simulink model "toma_datos"  (R2023a)
settings: Solver=VariableStepAuto  StartTime=0.0  StopTime=10.0  RelTol=1e-3
libraries: daqlib x2
settings Model: Creator=Juan  LastModifiedBy=Juan

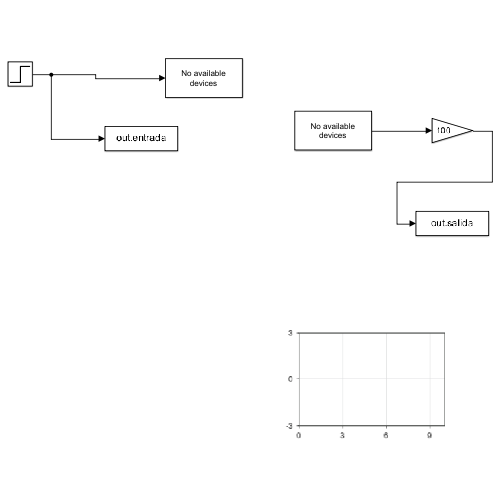
[thumbnail: Simulink's stored preview of the top-level diagram]
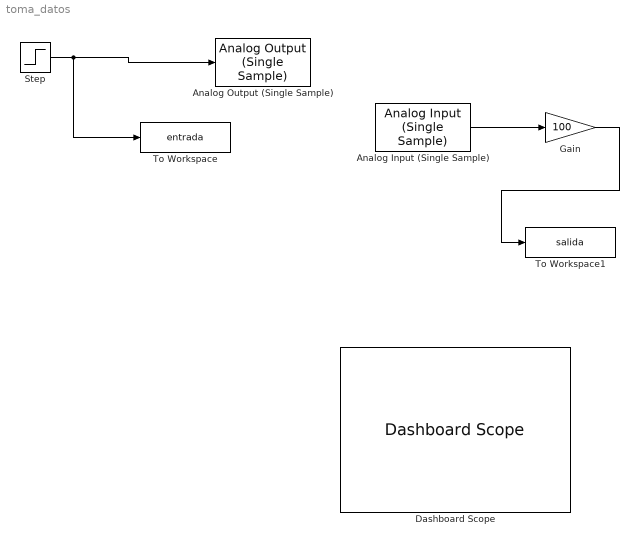
== system toma_datos ==
  Analog Input (Single Sample) : daqlib/Analog Input (Single Sample)  DeviceMenu=(none)  Device=(none)  BlockSampleTime=1  NChannelsSelected=1  NPorts=1 for all channels  OutputTimestamp=off
  Analog Output (Single Sample) : daqlib/Analog Output (Single Sample)  DeviceMenu=(none)  Device=(none)  NChannelsSelected=1  NPorts=1 for all channels  BlockSampleTime=1
  Dashboard Scope : DashboardScope
  Gain : Gain  Gain=100
  Step : Step  Time=0  After=5  SampleTime=0
  To Workspace : ToWorkspace  VariableName=entrada  SaveFormat=Timeseries  SampleTime=-1
  To Workspace1 : ToWorkspace  VariableName=salida  SaveFormat=Timeseries  SampleTime=-1
  wires:
  Step/1 -> To Workspace/1, Analog Output (Single Sample)/1
  Analog Input (Single Sample)/1 -> Gain/1
  Gain/1 -> To Workspace1/1
